simulink library "AMK_model_lib"  (R2022b)
settings: Solver=VariableStepAuto  StartTime=0.0  StopTime=10.0  RelTol=1e-3
undefined symbols (not defined in the file): DiscIntNeverNeededParam
libraries: $bdroot x15, AMK_CAN_lib x6, dspstat3 x1, slpidlib x1, simulink x1
settings Model: Creator=dr_pa  LastModifiedBy=dr_pa

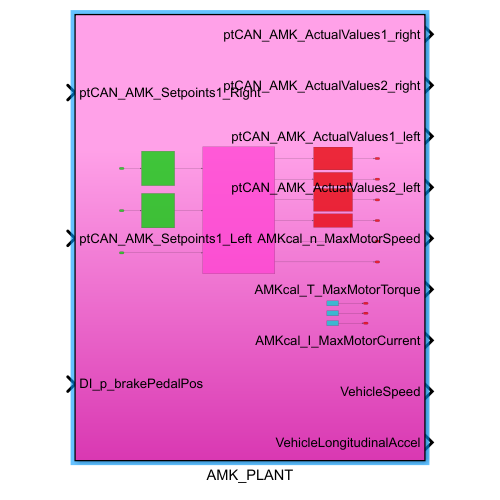
[thumbnail: Simulink's stored preview of the top-level diagram]
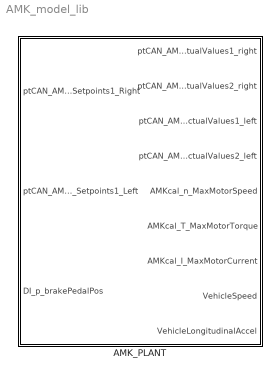
== system AMK_model_lib ==
  AMK_PLANT : Subsystem

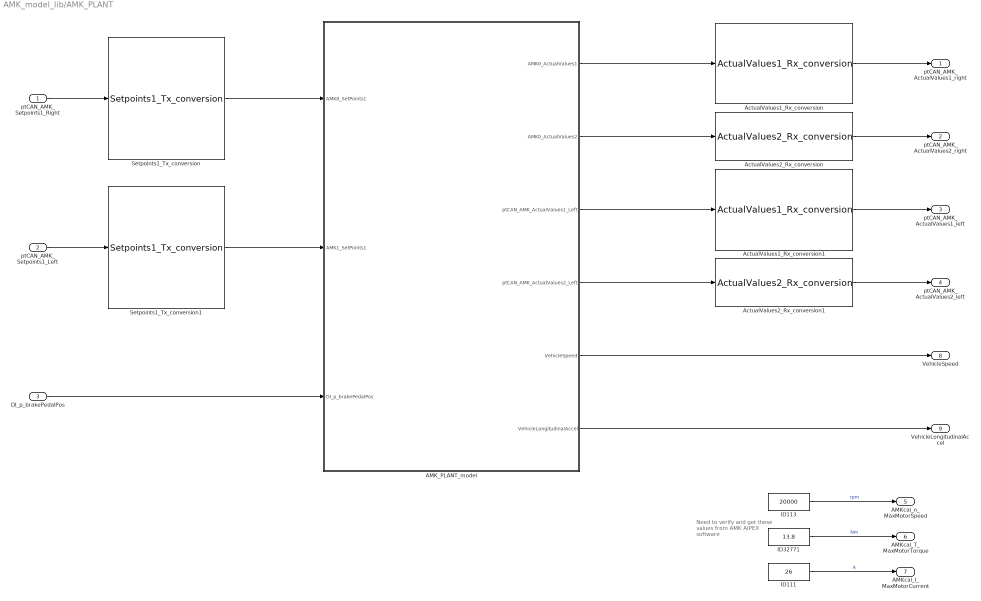
== system AMK_model_lib/AMK_PLANT ==
  note: Need to verify and get
      | these values from AMK
      | AIPEX software
  ptCAN_AMK_Setpoints1_Right : Inport
  ptCAN_AMK_Setpoints1_Left : Inport  Port=2
  DI_p_brakePedalPos : Inport  Port=3
  AMK_PLANT_model : Subsystem
  ActualValues1_Rx_conversion : AMK_CAN_lib/AMK_CAN/ActualValues1_Rx_conversion  SystemSampleTime=-1  VariantActivationTime=update diagram  Latency=0  AutoFrameSizeCalculation=off
  ActualValues1_Rx_conversion1 : AMK_CAN_lib/AMK_CAN/ActualValues1_Rx_conversion  SystemSampleTime=-1  VariantActivationTime=update diagram  Latency=0  AutoFrameSizeCalculation=off
  ActualValues2_Rx_conversion : AMK_CAN_lib/AMK_CAN/ActualValues2_Rx_conversion  SystemSampleTime=-1  VariantActivationTime=update diagram  Latency=0  AutoFrameSizeCalculation=off
  ActualValues2_Rx_conversion1 : AMK_CAN_lib/AMK_CAN/ActualValues2_Rx_conversion  SystemSampleTime=-1  VariantActivationTime=update diagram  Latency=0  AutoFrameSizeCalculation=off
  ID111 : Constant  Value=26  OutDataTypeStr=single
  ID113 : Constant  Value=20000  OutDataTypeStr=single
  ID32771 : Constant  Value=13.8  OutDataTypeStr=single
  Setpoints1_Tx_conversion : AMK_CAN_lib/AMK_CAN/Setpoints1_Tx_conversion  SystemSampleTime=-1  VariantActivationTime=update diagram  Latency=0  AutoFrameSizeCalculation=off
  Setpoints1_Tx_conversion1 : AMK_CAN_lib/AMK_CAN/Setpoints1_Tx_conversion  SystemSampleTime=-1  VariantActivationTime=update diagram  Latency=0  AutoFrameSizeCalculation=off
  ptCAN_AMK_ActualValues1_right : Outport
  ptCAN_AMK_ActualValues2_right : Outport  Port=2
  ptCAN_AMK_ActualValues1_left : Outport  Port=3
  ptCAN_AMK_ActualValues2_left : Outport  Port=4
  AMKcal_n_MaxMotorSpeed : Outport  Port=5
  AMKcal_T_MaxMotorTorque : Outport  Port=6
  AMKcal_I_MaxMotorCurrent : Outport  Port=7
  VehicleSpeed : Outport  Port=8
  VehicleLongitudinalAccel : Outport  Port=9
  wires:
  DI_p_brakePedalPos/1 -> AMK_PLANT_model/3(DI_p_brakePedalPos)
  AMK_PLANT_model/1(AMK0_ActualValues1) -> ActualValues1_Rx_conversion/1
  AMK_PLANT_model/2(AMK0_ActualValues2) -> ActualValues2_Rx_conversion/1
  AMK_PLANT_model/3(ptCAN_AMK_ActualValues1_Left) -> ActualValues1_Rx_conversion1/1
  AMK_PLANT_model/5(VehicleSpeed) -> VehicleSpeed/1
  AMK_PLANT_model/6(VehicleLongitudinalAccel) -> VehicleLongitudinalAccel/1
  Setpoints1_Tx_conversion/1 -> AMK_PLANT_model/1(AMK0_SetPoints1)
  ptCAN_AMK_Setpoints1_Right/1 -> Setpoints1_Tx_conversion/1
  Setpoints1_Tx_conversion1/1 -> AMK_PLANT_model/2(AMK1_SetPoints1)
  ptCAN_AMK_Setpoints1_Left/1 -> Setpoints1_Tx_conversion1/1
  AMK_PLANT_model/4(ptCAN_AMK_ActualValues2_Left) -> ActualValues2_Rx_conversion1/1
  ActualValues1_Rx_conversion/1 -> ptCAN_AMK_ActualValues1_right/1
  ActualValues2_Rx_conversion/1 -> ptCAN_AMK_ActualValues2_right/1
  ActualValues1_Rx_conversion1/1 -> ptCAN_AMK_ActualValues1_left/1
  ActualValues2_Rx_conversion1/1 -> ptCAN_AMK_ActualValues2_left/1
  ID113/1 -> AMKcal_n_MaxMotorSpeed/1  "rpm"
  ID32771/1 -> AMKcal_T_MaxMotorTorque/1  "Nm"
  ID111/1 -> AMKcal_I_MaxMotorCurrent/1  "A"

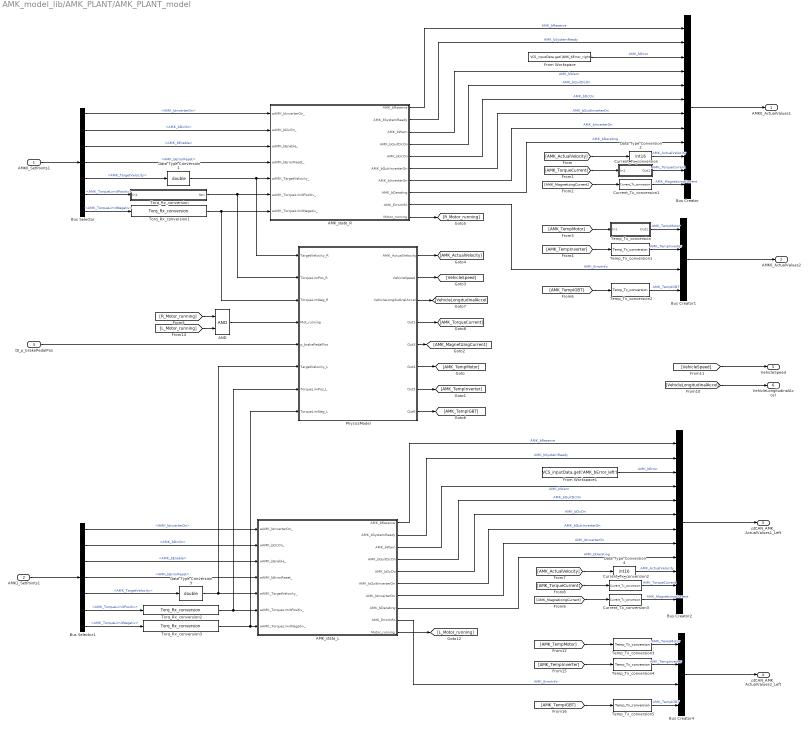
== system AMK_model_lib/AMK_PLANT/AMK_PLANT_model ==
  AMK0_SetPoints1 : Inport
  AMK1_SetPoints1 : Inport  Port=2
  DI_p_brakePedalPos : Inport  Port=3
  AMK_state_L : Stateflow chart  TreatAsAtomicUnit=on
  AMK_state_R : Stateflow chart  TreatAsAtomicUnit=on
  AND : Logic  IconShape=distinctive  AllPortsSameDT=off  OutDataTypeStr=boolean
  Bus Creator : BusCreator  Inputs=12
  Bus Creator1 : BusCreator  Inputs=4
  Bus Creator2 : BusCreator  Inputs=12
  Bus Creator4 : BusCreator  Inputs=4
  Bus Selector : BusSelector  OutputSignals=AMK_bInverterOn,AMK_bDcOn,AMK_bEnable,AMK_bErrorReset,AMK_TargetVelocity,AMK_TorqueLimitPositiv,AMK_TorqueLimitNegativ
  Bus Selector1 : BusSelector  OutputSignals=AMK_bInverterOn,AMK_bDcOn,AMK_bEnable,AMK_bErrorReset,AMK_TargetVelocity,AMK_TorqueLimitPositiv,AMK_TorqueLimitNegativ
  Current_Tx_conversion : Subsystem
  Current_Tx_conversion1 : $bdroot/AMK_PLANT/AMK_PLANT_model/Current_Tx_conversion  SystemSampleTime=-1  VariantActivationTime=update diagram  Latency=0  AutoFrameSizeCalculation=off
  Current_Tx_conversion2 : $bdroot/AMK_PLANT/AMK_PLANT_model/Current_Tx_conversion  SystemSampleTime=-1  VariantActivationTime=update diagram  Latency=0  AutoFrameSizeCalculation=off
  Current_Tx_conversion3 : $bdroot/AMK_PLANT/AMK_PLANT_model/Current_Tx_conversion  SystemSampleTime=-1  VariantActivationTime=update diagram  Latency=0  AutoFrameSizeCalculation=off
  Data Type Conversion1 : DataTypeConversion  OutDataTypeStr=double  SaturateOnIntegerOverflow=off  RndMeth=Floor
  Data Type Conversion2 : DataTypeConversion  OutDataTypeStr=int16  SaturateOnIntegerOverflow=off  RndMeth=Floor
  Data Type Conversion3 : DataTypeConversion  OutDataTypeStr=double  SaturateOnIntegerOverflow=off  RndMeth=Floor
  Data Type Conversion4 : DataTypeConversion  OutDataTypeStr=int16  SaturateOnIntegerOverflow=off  RndMeth=Floor
  From Workspace : FromWorkspace  VariableName=VCS_inputData.get('AMK_bError_right')
  From Workspace1 : FromWorkspace  VariableName=VCS_inputData.get('AMK_bError_left')
  PhysicsModel : Subsystem
  Temp_Tx_conversion : Subsystem
  Temp_Tx_conversion{1..5} (5 alike) : $bdroot/AMK_PLANT/AMK_PLANT_model/Temp_Tx_conversion  SystemSampleTime=-1  VariantActivationTime=update diagram  Latency=0  AutoFrameSizeCalculation=off
  Torq_Rx_conversion : Subsystem
  Torq_Rx_conversion1 : $bdroot/AMK_PLANT/AMK_PLANT_model/Torq_Rx_conversion  SystemSampleTime=-1  VariantActivationTime=update diagram  Latency=0  AutoFrameSizeCalculation=off
  Torq_Rx_conversion2 : $bdroot/AMK_PLANT/AMK_PLANT_model/Torq_Rx_conversion  SystemSampleTime=-1  VariantActivationTime=update diagram  Latency=0  AutoFrameSizeCalculation=off
  Torq_Rx_conversion3 : $bdroot/AMK_PLANT/AMK_PLANT_model/Torq_Rx_conversion  SystemSampleTime=-1  VariantActivationTime=update diagram  Latency=0  AutoFrameSizeCalculation=off
  AMK0_ActualValues1 : Outport
  AMK0_ActualValues2 : Outport  Port=2
  ptCAN_AMK_ActualValues1_Left : Outport  Port=3
  ptCAN_AMK_ActualValues2_Left : Outport  Port=4
  VehicleSpeed : Outport  Port=5
  VehicleLongitudinalAccel : Outport  Port=6
  wires:
  Bus Creator2/1 -> ptCAN_AMK_ActualValues1_Left/1
  Bus Creator/1 -> AMK0_ActualValues1/1
  AMK_state_R/3(AMK_bWarn) -> Bus Creator/4  "AMK_bWarn"
  Temp_Tx_conversion1/1 -> Bus Creator1/2  "AMK_TempInverter"
  PhysicsModel/1(AMK_ActualVelocity) -> [AMK_ActualVelocity]
  Data Type Conversion1/1 -> PhysicsModel/1(TargetVelocity_R), AMK_state_R/5(aAMK_TargetVelocity_)
  AMK1_SetPoints1/1 -> Bus Selector1/1
  [R_Motor_running] -> AND/1
  Current_Tx_conversion/1(Out1) -> Bus Creator/11  "AMK_TorqueCurrent"
  Data Type Conversion3/1 -> AMK_state_L/5(aAMK_TargetVelocity_), PhysicsModel/6(TargetVelocity_L)
  AMK_state_L/2(AMK_bSystemReady) -> Bus Creator2/2  "AMK_bSystemReady"
  PhysicsModel/7(Out5) -> [AMK_TempInverter]
  Current_Tx_conversion1/1 -> Bus Creator/12  "AMK_MagnetizingCurrent"
  Bus Creator4/1 -> ptCAN_AMK_ActualValues2_Left/1
  From Workspace/1 -> Bus Creator/3  "AMK_bError"
  AMK_state_R/9(AMK_ErrorInfo) -> Bus Creator1/3  "AMK_ErrorInfo"
  [AMK_TorqueCurrent] -> Current_Tx_conversion/1(In1)
  AMK_state_R/6(AMK_bQuitInverterOn) -> Bus Creator/7  "AMK_bQuitInverterOn"
  AMK_state_R/5(AMK_bDcOn) -> Bus Creator/6  "AMK_bDcOn"
  AMK_state_L/4(AMK_bQuitDcOn) -> Bus Creator2/5  "AMK_bQuitDcOn"
  AMK_state_R/10(Motor_running) -> [R_Motor_running]
  From Workspace1/1 -> Bus Creator2/3  "AMK_bError"
  PhysicsModel/2(VehicleSpeed) -> [VehicleSpeed]
  Bus Selector/3 -> AMK_state_R/3(aAMK_bEnable_)  "<AMK_bEnable>"
  AMK_state_R/8(AMK_bDerating) -> Bus Creator/9  "AMK_bDerating"
  Bus Selector/5 -> Data Type Conversion1/1  "<AMK_TargetVelocity>"
  [AMK_ActualVelocity] -> Data Type Conversion2/1
  AMK_state_L/10(Motor_running) -> [L_Motor_running]
  Torq_Rx_conversion1/1 -> PhysicsModel/3(TorqueLimNeg_R), AMK_state_R/7(aAMK_TorqueLimitNegativ_)
  Torq_Rx_conversion2/1 -> AMK_state_L/6(aAMK_TorqueLimitPositiv_), PhysicsModel/7(TorqueLimPos_L)
  AMK_state_L/5(AMK_bDcOn) -> Bus Creator2/6  "AMK_bDcOn"
  AND/1 -> PhysicsModel/4(Mot_running)
  Bus Creator1/1 -> AMK0_ActualValues2/1
  AMK_state_R/7(AMK_bInverterOn) -> Bus Creator/8  "AMK_bInverterOn"
  PhysicsModel/4(Out1) -> [AMK_TorqueCurrent]
  AMK_state_L/6(AMK_bQuitInverterOn) -> Bus Creator2/7  "AMK_bQuitInverterOn"
  Bus Selector1/1 -> AMK_state_L/1(aAMK_bInverterOn_)  "<AMK_bInverterOn>"
  PhysicsModel/8(Out6) -> [AMK_TempIGBT]
  AMK_state_L/9(AMK_ErrorInfo) -> Bus Creator4/3  "AMK_ErrorInfo"
  AMK_state_L/1(AMK_bReserve) -> Bus Creator2/1  "AMK_bReserve"
  Torq_Rx_conversion/1(Nm) -> PhysicsModel/2(TorqueLimPos_R), AMK_state_R/6(aAMK_TorqueLimitPositiv_)
  Bus Selector/2 -> AMK_state_R/2(aAMK_bDcOn_)  "<AMK_bDcOn>"
  Bus Selector1/3 -> AMK_state_L/3(aAMK_bEnable_)  "<AMK_bEnable>"
  Bus Selector1/4 -> AMK_state_L/4(aAMK_bErrorReset_)  "<AMK_bErrorReset>"
  AMK_state_L/3(AMK_bWarn) -> Bus Creator2/4  "AMK_bWarn"
  PhysicsModel/5(Out3) -> [AMK_MagnetizingCurrent]
  [L_Motor_running] -> AND/2
  DI_p_brakePedalPos/1 -> PhysicsModel/5(p_brakePedalPos)
  AMK_state_R/1(AMK_bReserve) -> Bus Creator/1  "AMK_bReserve"
  Temp_Tx_conversion/1(Out1) -> Bus Creator1/1  "AMK_TempMotor"
  Bus Selector1/5 -> Data Type Conversion3/1  "<AMK_TargetVelocity>"
  Torq_Rx_conversion3/1 -> AMK_state_L/7(aAMK_TorqueLimitNegativ_), PhysicsModel/8(TorqueLimNeg_L)
  PhysicsModel/3(VehicleLongitudinalAccel) -> [VehicleLongitudinalAccel]
  PhysicsModel/6(Out4) -> [AMK_TempMotor]
  Current_Tx_conversion3/1 -> Bus Creator2/12  "AMK_MagnetizingCurrent"
  [VehicleLongitudinalAccel] -> VehicleLongitudinalAccel/1
  Current_Tx_conversion2/1 -> Bus Creator2/11  "AMK_TorqueCurrent"
  Data Type Conversion4/1 -> Bus Creator2/10  "AMK_ActualVelocity"
  Temp_Tx_conversion2/1 -> Bus Creator1/4  "AMK_TempIGBT"
  Data Type Conversion2/1 -> Bus Creator/10  "AMK_ActualVelocity"
  [AMK_MagnetizingCurrent] -> Current_Tx_conversion1/1
  Temp_Tx_conversion3/1 -> Bus Creator4/1  "AMK_TempMotor"
  Bus Selector/4 -> AMK_state_R/4(aAMK_bErrorReset_)  "<AMK_bErrorReset>"
  AMK_state_L/8(AMK_bDerating) -> Bus Creator2/9  "AMK_bDerating"
  AMK_state_R/4(AMK_bQuitDcOn) -> Bus Creator/5  "AMK_bQuitDcOn"
  Bus Selector/1 -> AMK_state_R/1(aAMK_bInverterOn_)  "<AMK_bInverterOn>"
  Bus Selector1/2 -> AMK_state_L/2(aAMK_bDcOn_)  "<AMK_bDcOn>"
  AMK0_SetPoints1/1 -> Bus Selector/1
  Temp_Tx_conversion4/1 -> Bus Creator4/2  "AMK_TempInverter"
  AMK_state_L/7(AMK_bInverterOn) -> Bus Creator2/8  "AMK_bInverterOn"
  Temp_Tx_conversion5/1 -> Bus Creator4/4  "AMK_TempIGBT"
  AMK_state_R/2(AMK_bSystemReady) -> Bus Creator/2  "AMK_bSystemReady"
  [VehicleSpeed] -> VehicleSpeed/1
  Bus Selector/6 -> Torq_Rx_conversion/1(In1)  "<AMK_TorqueLimitPositiv>"
  Bus Selector/7 -> Torq_Rx_conversion1/1  "<AMK_TorqueLimitNegativ>"
  ? -> ?  "<AMK_TargetVelocity>"
  Bus Selector1/6 -> Torq_Rx_conversion2/1  "<AMK_TorqueLimitPositiv>"
  Bus Selector1/7 -> Torq_Rx_conversion3/1  "<AMK_TorqueLimitNegativ>"
  [AMK_TempMotor] -> Temp_Tx_conversion/1(In1)
  [AMK_TempInverter] -> Temp_Tx_conversion1/1
  [AMK_TempIGBT] -> Temp_Tx_conversion2/1
  [AMK_TempMotor] -> Temp_Tx_conversion3/1
  [AMK_TempInverter] -> Temp_Tx_conversion4/1
  [AMK_TempIGBT] -> Temp_Tx_conversion5/1
  [AMK_ActualVelocity] -> Data Type Conversion4/1
  [AMK_TorqueCurrent] -> Current_Tx_conversion2/1
  [AMK_MagnetizingCurrent] -> Current_Tx_conversion3/1

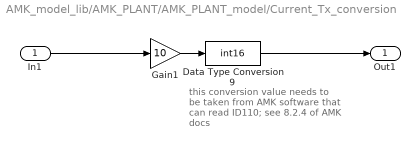
== system AMK_model_lib/AMK_PLANT/AMK_PLANT_model/Current_Tx_conversion ==
  note: this conversion value needs to be taken from AMK software that can read ID110; see 8.2.4 of AMK docs
  In1 : Inport
  Data Type Conversion9 : DataTypeConversion  OutDataTypeStr=int16  SaturateOnIntegerOverflow=off  RndMeth=Floor
  Gain1 : Gain  Gain=10
  Out1 : Outport
  wires:
  Gain1/1 -> Data Type Conversion9/1
  Data Type Conversion9/1 -> Out1/1
  In1/1 -> Gain1/1

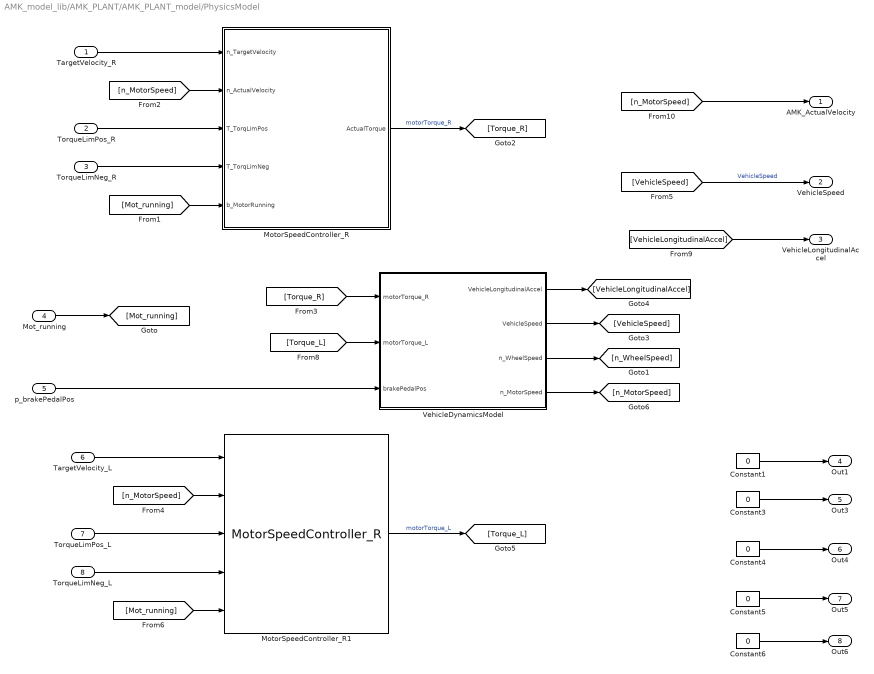
== system AMK_model_lib/AMK_PLANT/AMK_PLANT_model/PhysicsModel ==
  TargetVelocity_R : Inport
  TorqueLimPos_R : Inport  Port=2
  TorqueLimNeg_R : Inport  Port=3
  Mot_running : Inport  Port=4
  p_brakePedalPos : Inport  Port=5
  TargetVelocity_L : Inport  Port=6
  TorqueLimPos_L : Inport  Port=7
  TorqueLimNeg_L : Inport  Port=8
  Constant{1,3..6} (5 alike) : Constant  Value=0  OutDataTypeStr=single
  MotorSpeedController_R : Subsystem
  MotorSpeedController_R1 : $bdroot/AMK_PLANT/AMK_PLANT_model/PhysicsModel/MotorSpeedController_R  SystemSampleTime=-1  VariantActivationTime=update diagram  Latency=0  AutoFrameSizeCalculation=off
  VehicleDynamicsModel : Subsystem
  AMK_ActualVelocity : Outport
  VehicleSpeed : Outport  Port=2
  VehicleLongitudinalAccel : Outport  Port=3
  Out1 : Outport  Port=4
  Out3 : Outport  Port=5
  Out4 : Outport  Port=6
  Out5 : Outport  Port=7
  Out6 : Outport  Port=8
  wires:
  Mot_running/1 -> [Mot_running]
  [VehicleSpeed] -> VehicleSpeed/1  "VehicleSpeed"
  Constant3/1 -> Out3/1
  Constant4/1 -> Out4/1
  Constant5/1 -> Out5/1
  Constant6/1 -> Out6/1
  TargetVelocity_R/1 -> MotorSpeedController_R/1(n_TargetVelocity)
  TorqueLimPos_R/1 -> MotorSpeedController_R/3(T_TorqLimPos)
  TorqueLimNeg_R/1 -> MotorSpeedController_R/4(T_TorqLimNeg)
  [Mot_running] -> MotorSpeedController_R/5(b_MotorRunning)
  VehicleDynamicsModel/3(n_WheelSpeed) -> [n_WheelSpeed]
  [n_MotorSpeed] -> MotorSpeedController_R/2(n_ActualVelocity)
  MotorSpeedController_R/1(ActualTorque) -> [Torque_R]  "motorTorque_R"
  [Torque_R] -> VehicleDynamicsModel/1(motorTorque_R)
  [n_MotorSpeed] -> AMK_ActualVelocity/1
  VehicleDynamicsModel/2(VehicleSpeed) -> [VehicleSpeed]
  p_brakePedalPos/1 -> VehicleDynamicsModel/3(brakePedalPos)
  VehicleDynamicsModel/1(VehicleLongitudinalAccel) -> [VehicleLongitudinalAccel]
  MotorSpeedController_R1/1 -> [Torque_L]  "motorTorque_L"
  [n_MotorSpeed] -> MotorSpeedController_R1/2
  [Mot_running] -> MotorSpeedController_R1/5
  TorqueLimNeg_L/1 -> MotorSpeedController_R1/4
  TorqueLimPos_L/1 -> MotorSpeedController_R1/3
  TargetVelocity_L/1 -> MotorSpeedController_R1/1
  [Torque_L] -> VehicleDynamicsModel/2(motorTorque_L)
  [VehicleLongitudinalAccel] -> VehicleLongitudinalAccel/1
  VehicleDynamicsModel/4(n_MotorSpeed) -> [n_MotorSpeed]
  Constant1/1 -> Out1/1

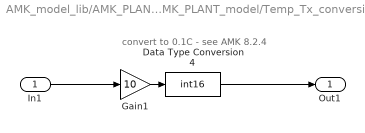
== system AMK_model_lib/AMK_PLANT/AMK_PLANT_model/Temp_Tx_conversion ==
  note: convert to 0.1C - see AMK 8.2.4
  In1 : Inport
  Data Type Conversion4 : DataTypeConversion  OutDataTypeStr=int16  SaturateOnIntegerOverflow=off  RndMeth=Floor
  Gain1 : Gain  Gain=10
  Out1 : Outport
  wires:
  Gain1/1 -> Data Type Conversion4/1
  In1/1 -> Gain1/1
  Data Type Conversion4/1 -> Out1/1

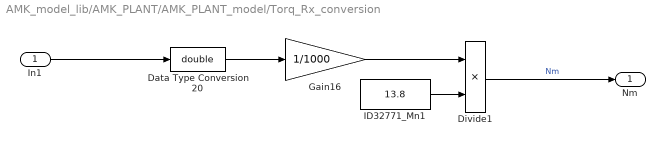
== system AMK_model_lib/AMK_PLANT/AMK_PLANT_model/Torq_Rx_conversion ==
  In1 : Inport
  Data Type Conversion20 : DataTypeConversion  OutDataTypeStr=double  SaturateOnIntegerOverflow=off  RndMeth=Floor
  Divide1 : Product  Inputs=**
  Gain16 : Gain  Gain=1/1000
  ID32771_Mn1 : Constant  Value=13.8  OutDataTypeStr=single
  Nm : Outport
  wires:
  ID32771_Mn1/1 -> Divide1/2
  Data Type Conversion20/1 -> Gain16/1
  Divide1/1 -> Nm/1  "Nm"
  Gain16/1 -> Divide1/1
  In1/1 -> Data Type Conversion20/1

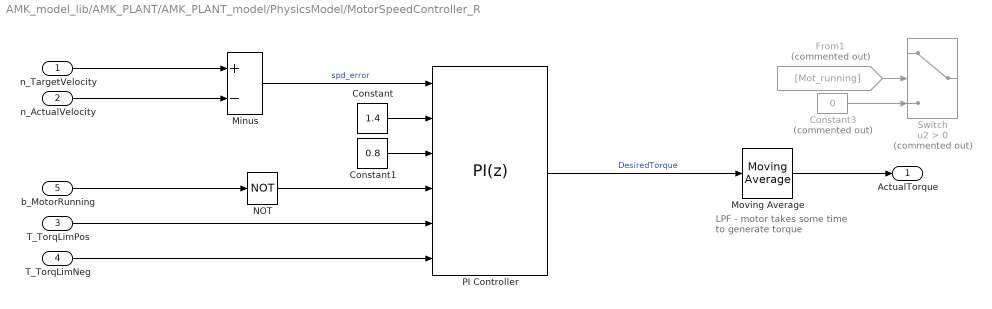
== system AMK_model_lib/AMK_PLANT/AMK_PLANT_model/PhysicsModel/MotorSpeedController_R ==
  note: LPF - motor takes some
      | time to generate torque
  n_TargetVelocity : Inport
  n_ActualVelocity : Inport  Port=2
  T_TorqLimPos : Inport  Port=3
  T_TorqLimNeg : Inport  Port=4
  b_MotorRunning : Inport  Port=5
  Constant : Constant  Value=1.4  OutDataTypeStr=single
  Constant1 : Constant  Value=0.8  OutDataTypeStr=single
  Constant3 : Constant  Commented=on  Value=0
  From1 : From  Commented=on  GotoTag=Mot_running
  Minus : Sum  Inputs=+-
  Moving Average : dspstat3/Moving Average  Method=Sliding window  ForgettingFactorPort=off  SpecifyWindowLength=on  WindowLength=5  OverlapLength=4  AllowArbitraryInputLength=off  ForgettingFactor=0.9  SimulateUsing=Code generation
  NOT : Logic  Operator=NOT  IconShape=distinctive  AllPortsSameDT=off  OutDataTypeStr=boolean
  PI Controller : slpidlib/PID Controller  Controller=PI  Form=Parallel  TimeDomain=Discrete-time  UseExternalTs=off  SampleTime=-1  IntegratorMethod=Forward Euler  FilterMethod=Forward Euler  ControllerParametersSource=external  P=1  I=1  UseKiTs=off  D=0  N=100  UseFilter=on  TunerSelectOption=Transfer Function Based (PID Tuner App)  InitialConditionSource=internal  InitialConditionForIntegrator=0  InitialConditionForFilter=0  DifferentiatorICPrevScaledInput=0  ExternalReset=level  TrackingMode=off  Kt=1  LimitOutput=on  SatLimitsSource=external  UpperSaturationLimit=1  LowerSaturationLimit=-1  LinearizeAsGain=on  AntiWindupMode=clamping  Kb=1  LimitIntegrator=off  UpperIntegratorSaturationLimit=inf  LowerIntegratorSaturationLimit=-inf  RndMeth=Simplest  POutMin=[]  POutMax=[]  IOutMin=[]  IOutMax=[]  DOutMin=[]  DOutMax=[]  NOutMin=[]  NOutMax=[]  SumOutMin=[]  SumOutMax=[]  SaturationOutDataTypeStr=single  SaturationOutMin=[]  SaturationOutMax=[]  PParamMin=[]  PParamMax=[]  IParamMin=[]  IParamMax=[]  DParamMin=[]  DParamMax=[]  NParamMin=[]  NParamMax=[]  KbParamMin=[]  KbParamMax=[]  KtParamMin=[]  KtParamMax=[]  KbOutMin=[]  KbOutMax=[]  KtOutMin=[]  KtOutMax=[]  IntegratorOutMin=[]  IntegratorOutMax=[]  FilterOutMin=[]  FilterOutMax=[]  SumI1OutMin=[]  SumI1OutMax=[]  SumI2OutMin=[]  SumI2OutMax=[]  SumI3OutMin=[]  SumI3OutMax=[]  SumI4OutMin=[]  SumI4OutMax=[]  SumDOutMin=[]  SumDOutMax=[]  DifferentiatorOutMin=[]  DifferentiatorOutMax=[]  FilterDiffOutCoefMin=[]  FilterDiffOutCoefMax=[]  ReciprocalOutMin=[]  ReciprocalOutMax=[]  SumDenOutMin=[]  SumDenOutMax=[]  SumNumOutMin=[]  SumNumOutMax=[]  DivideOutMin=[]  DivideOutMax=[]  UdiffTsProdOutMin=[]  UdiffTsProdOutMax=[]  NTsProdOutMin=[]  NTsProdOutMax=[]  UintegralTsProdOutMin=[]  UintegralTsProdOutMax=[]  UngainTsProdOutMin=[]  UngainTsProdOutMax=[]  ClampingZeroOutDataTypeStr=Inherit: Inherit via back propagation  ClampingZeroOutMin=[]  ClampingZeroOutMax=[]  FilterDenConstantOutDataTypeStr=Inherit: Inherit via back propagation  FilterDenConstantOutMin=[]  FilterDenConstantOutMax=[]  PCopyOutDataTypeStr=Inherit: Inherit via back propagation  PCopyOutMin=[]  PCopyOutMax=[]  NCopyOutDataTypeStr=Inherit: Inherit via back propagation  NCopyOutMin=[]  NCopyOutMax=[]  IntegratorContinuousStateAttributes=''  IntegratorStateMustResolveToSignalObject=off  IntegratorRTWStateStorageClass=Auto  FilterContinuousStateAttributes=''  FilterStateMustResolveToSignalObject=off  FilterRTWStateStorageClass=Auto  ParallelPVariant=ExternalParameters  IdealPVariant=Disabled  IVariant=ExternalParameters  DVariant=Disabled  IntegratorVariant=Discrete  SatVariant=External  AWVariant=DiscClampingParallel  PCopyVariant=Disabled  TRVariant=Disabled  FdbkBlocksVariant=Forward  IdealPFdbkVariant=Disabled  SatFdbkVariant=Disabled  DerivativeFilterVariant=Disabled  NVariant=Disabled  NCopyVariant=Disabled_SignalSpec  FilterICVariant=Disabled  IntegratorICVariant=InternalICs  ExternalResetVariant=ExternalReset  TRSumVariant=Passthrough  SumFdbkVariant=Disabled  SumVariant=Sum_PI  TsampFilterVariant=InternalTs  TsampNgainVariant=Passthrough  TsampIntegralVariant=Passthrough  ExternalSaturationOutDataTypeStr=single
      settings: LibrarySourceBlock=mcbhdllib/Controls/Controllers/PI Controller
  Switch : Switch  Commented=on  Criteria=u2 > Threshold  OutDataTypeStr=single  SaturateOnIntegerOverflow=off  InputSameDT=off
  ActualTorque : Outport
  wires:
  NOT/1 -> PI Controller/4
  b_MotorRunning/1 -> NOT/1
  T_TorqLimNeg/1 -> PI Controller/6
  Minus/1 -> PI Controller/1  "spd_error"
  n_TargetVelocity/1 -> Minus/1
  PI Controller/1 -> Moving Average/1  "DesiredTorque"
  Constant/1 -> PI Controller/2
  Constant1/1 -> PI Controller/3
  n_ActualVelocity/1 -> Minus/2
  From1/1 -> Switch/2
  Constant3/1 -> Switch/3
  Moving Average/1 -> ActualTorque/1
  T_TorqLimPos/1 -> PI Controller/5

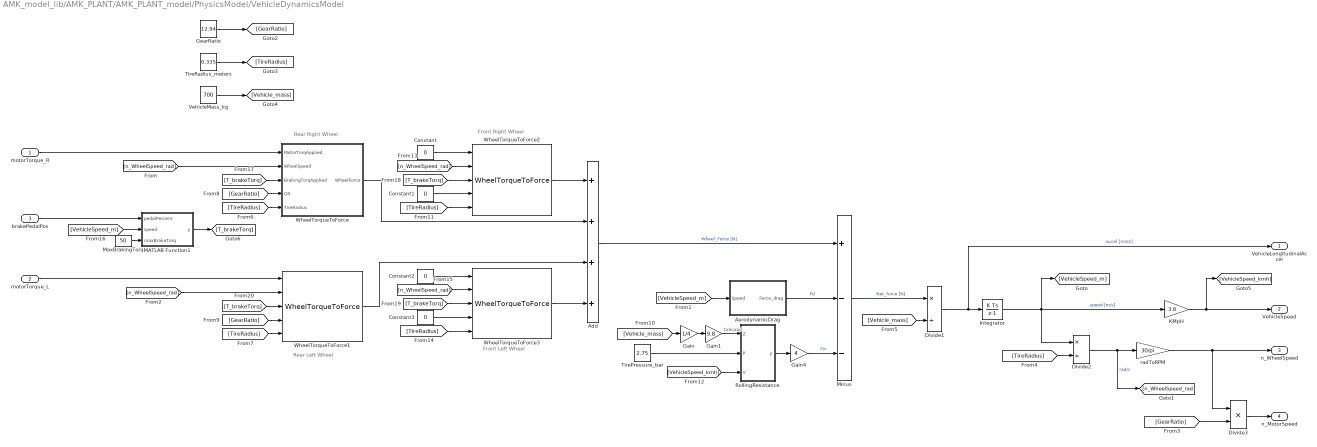
== system AMK_model_lib/AMK_PLANT/AMK_PLANT_model/PhysicsModel/VehicleDynamicsModel ==
  note: Rear Right Wheel
  note: Rear Left Wheel
  note: Front Right Wheel
  note: Front Left Wheel
  motorTorque_R : Inport
  motorTorque_L : Inport  Port=2
  brakePedalPos : Inport  Port=3
  Add : Sum  Inputs=++++
  AerodynamicDrag : Subsystem
  Constant{,1..3} (4 alike) : Constant  Value=0  OutDataTypeStr=single
  Divide1 : Product  Inputs=*/
  Divide2 : Product  Inputs=*/
  Divide3 : Product  Inputs=**
  Gain : Gain  Gain=1/4
  Gain1 : Gain  Gain=9.8
  Gain4 : Gain  Gain=4
  GearRatio : Constant  Value=12.94  OutDataTypeStr=single
  Integrator : DiscreteIntegrator  SampleTime=-1  ICPrevOutput=DiscIntNeverNeededParam  ICPrevScaledInput=DiscIntNeverNeededParam
  KMpH : Gain  Gain=3.6
  MATLAB Function1 : MATLAB Function  TreatAsAtomicUnit=on
  MaxBrakingTorq : Constant  Value=50  OutDataTypeStr=single
  Minus : Sum  Inputs=+--
  RollingResistance : MATLAB Function  TreatAsAtomicUnit=on
  TirePressure_bar : Constant  Value=2.75  OutDataTypeStr=single
  TireRadius_meters : Constant  Value=0.335  OutDataTypeStr=single
  VehicleMass_kg : Constant  Value=700  OutDataTypeStr=single
  WheelTorqueToForce : Subsystem
  WheelTorqueToForce1 : $bdroot/AMK_PLANT/AMK_PLANT_model/PhysicsModel/VehicleDynamicsModel/WheelTorqueToForce  SystemSampleTime=-1  VariantActivationTime=update diagram  Latency=0  AutoFrameSizeCalculation=off
  WheelTorqueToForce2 : $bdroot/AMK_PLANT/AMK_PLANT_model/PhysicsModel/VehicleDynamicsModel/WheelTorqueToForce  SystemSampleTime=-1  VariantActivationTime=update diagram  Latency=0  AutoFrameSizeCalculation=off
  WheelTorqueToForce3 : $bdroot/AMK_PLANT/AMK_PLANT_model/PhysicsModel/VehicleDynamicsModel/WheelTorqueToForce  SystemSampleTime=-1  VariantActivationTime=update diagram  Latency=0  AutoFrameSizeCalculation=off
  radToRPM : Gain  Gain=30/pi
  VehicleLongitudinalAccel : Outport
  VehicleSpeed : Outport  Port=2
  n_WheelSpeed : Outport  Port=3
  n_MotorSpeed : Outport  Port=4
  wires:
  radToRPM/1 -> Divide3/1, n_WheelSpeed/1
  motorTorque_R/1 -> WheelTorqueToForce/1(MotorTorqApplied)
  [n_WheelSpeed_rad] -> WheelTorqueToForce/2(WheelSpeed)
  Add/1 -> Minus/1  "Wheel_Force [N]"
  [n_WheelSpeed_rad] -> WheelTorqueToForce1/2
  motorTorque_L/1 -> WheelTorqueToForce1/1
  brakePedalPos/1 -> MATLAB Function1/1(pedalPercent)
  MaxBrakingTorq/1 -> MATLAB Function1/3(maxBrakeTorq)
  Divide1/1 -> Integrator/1, VehicleLongitudinalAccel/1  "accel [m/s2]"
  Integrator/1 -> Divide2/1, [VehicleSpeed_m], KMpH/1  "speed [m/s]"
  KMpH/1 -> [VehicleSpeed_kmh], VehicleSpeed/1
  Divide2/1 -> [n_WheelSpeed_rad], radToRPM/1  "rad/s"
  Minus/1 -> Divide1/1  "Net_force [N]"
  [VehicleSpeed_m] -> AerodynamicDrag/1(Speed)
  AerodynamicDrag/1(Force_drag) -> Minus/2  "Fd"
  GearRatio/1 -> [GearRatio]
  Divide3/1 -> n_MotorSpeed/1
  [GearRatio] -> Divide3/2
  TireRadius_meters/1 -> [TireRadius]
  VehicleMass_kg/1 -> [Vehicle_mass]
  [TireRadius] -> Divide2/2
  [Vehicle_mass] -> Divide1/2
  [TireRadius] -> WheelTorqueToForce/5(TireRadius)
  [TireRadius] -> WheelTorqueToForce1/5
  [GearRatio] -> WheelTorqueToForce/4(GR)
  [GearRatio] -> WheelTorqueToForce1/4
  [VehicleSpeed_kmh] -> RollingResistance/3(V)
  [Vehicle_mass] -> Gain/1
  Gain/1 -> Gain1/1
  Gain1/1 -> RollingResistance/1(Z)  "tireLoad"
  TirePressure_bar/1 -> RollingResistance/2(P)
  RollingResistance/1(y) -> Gain4/1
  Gain4/1 -> Minus/3  "Frr"
  Constant1/1 -> WheelTorqueToForce2/4
  WheelTorqueToForce2/1 -> Add/1
  WheelTorqueToForce/1(WheelForce) -> Add/2
  [TireRadius] -> WheelTorqueToForce2/5
  Constant/1 -> WheelTorqueToForce2/1
  [n_WheelSpeed_rad] -> WheelTorqueToForce2/2
  [TireRadius] -> WheelTorqueToForce3/5
  Constant2/1 -> WheelTorqueToForce3/1
  Constant3/1 -> WheelTorqueToForce3/4
  [n_WheelSpeed_rad] -> WheelTorqueToForce3/2
  [VehicleSpeed_m] -> MATLAB Function1/2(speed)
  WheelTorqueToForce3/1 -> Add/4
  WheelTorqueToForce1/1 -> Add/3
  MATLAB Function1/1(y) -> [T_brakeTorq]
  [T_brakeTorq] -> WheelTorqueToForce/3(BrakingTorqApplied)
  [T_brakeTorq] -> WheelTorqueToForce2/3
  [T_brakeTorq] -> WheelTorqueToForce3/3
  [T_brakeTorq] -> WheelTorqueToForce1/3

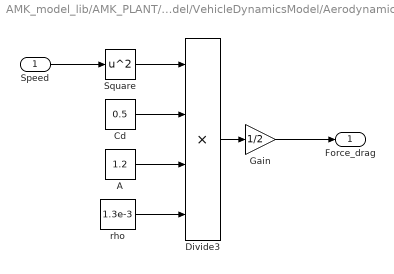
== system AMK_model_lib/AMK_PLANT/AMK_PLANT_model/PhysicsModel/VehicleDynamicsModel/AerodynamicDrag ==
  Speed : Inport
  A : Constant  Value=1.2  OutDataTypeStr=single
  Cd : Constant  Value=0.5  OutDataTypeStr=single
  Divide3 : Product  Inputs=****
  Gain : Gain  Gain=1/2
  Square : Math  Operator=square
  rho : Constant  Value=1.3e-3  OutDataTypeStr=single
  Force_drag : Outport
  wires:
  Gain/1 -> Force_drag/1
  rho/1 -> Divide3/4
  Divide3/1 -> Gain/1
  Square/1 -> Divide3/1
  A/1 -> Divide3/3
  Speed/1 -> Square/1
  Cd/1 -> Divide3/2

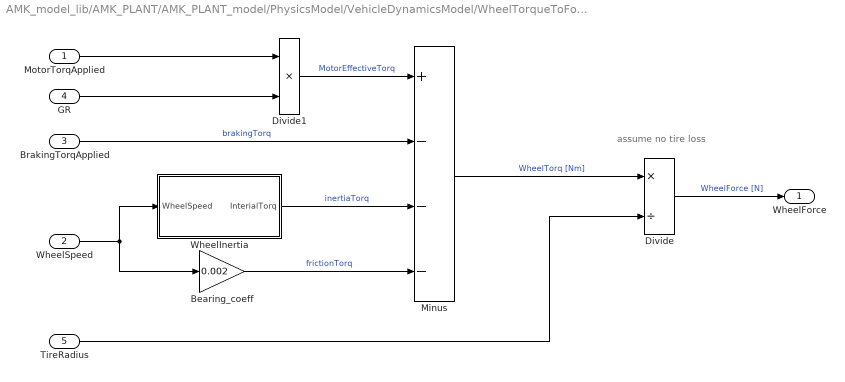
== system AMK_model_lib/AMK_PLANT/AMK_PLANT_model/PhysicsModel/VehicleDynamicsModel/WheelTorqueToForce ==
  note: assume no tire loss
  MotorTorqApplied : Inport
  WheelSpeed : Inport  Port=2
  BrakingTorqApplied : Inport  Port=3
  GR : Inport  Port=4
  TireRadius : Inport  Port=5
  Bearing_coeff : Gain  Gain=0.002
  Divide : Product  Inputs=*/
  Divide1 : Product  Inputs=**
  Minus : Sum  Inputs=+---
  WheelInertia : Subsystem
  WheelForce : Outport
  wires:
  WheelSpeed/1 -> WheelInertia/1(WheelSpeed), Bearing_coeff/1
  Minus/1 -> Divide/1  "WheelTorq [Nm]"
  WheelInertia/1(InterialTorq) -> Minus/3  "inertiaTorq"
  Divide1/1 -> Minus/1  "MotorEffectiveTorq"
  TireRadius/1 -> Divide/2
  Divide/1 -> WheelForce/1  "WheelForce [N]"
  MotorTorqApplied/1 -> Divide1/1
  BrakingTorqApplied/1 -> Minus/2  "brakingTorq"
  Bearing_coeff/1 -> Minus/4  "frictionTorq"
  GR/1 -> Divide1/2

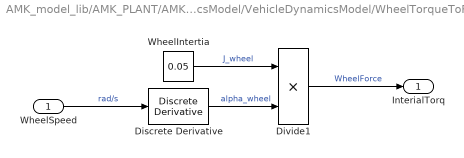
== system AMK_model_lib/AMK_PLANT/AMK_PLANT_model/PhysicsModel/VehicleDynamicsModel/WheelTorqueToForce/WheelInertia ==
  WheelSpeed : Inport
  Discrete Derivative : simulink/Discrete/Discrete Derivative  gainval=1.0  ICPrevScaledInput=0.0  OutMin=[]  OutMax=[]  OutDataType=fixdt(1, 16)  OutScaling=2^-10  DoSatur=off
  Divide1 : Product  Inputs=**
  WheelIntertia : Constant  Value=0.05  OutDataTypeStr=single
  InterialTorq : Outport
  wires:
  Discrete Derivative/1 -> Divide1/2  "alpha_wheel"
  Divide1/1 -> InterialTorq/1  "WheelForce"
  WheelSpeed/1 -> Discrete Derivative/1  "rad/s"
  WheelIntertia/1 -> Divide1/1  "J_wheel"

== stateflow chart AMK_model_lib/AMK_PLANT/AMK_PLANT_model/AMK_state_L ==
  state AMK_idle
    en:
    AMK_bReserve = 0;
    AMK_bSystemReady = 0;
    AMK_bWarn = 0;
    AMK_bQuitDcOn = 0;
    AMK_bDcOn = 0;
    AMK_bQuitInverterOn = 0;
    AMK_bInverterOn = 0;
    AMK_bDerating = 0;
    AMK_ErrorInfo = 0;
    Motor_running = false;
  note: Enable
      | en_
      | aAMK_bInverterOn_= 1
  state Startup [group]
    state Enable_System_Ready
      en:
      AMK_bSystemReady = 1;
    state Enable_Quit_Dc_On
      en:
      AMK_bQuitDcOn = 1;
      AMK_bDcOn = 1;
    state Inverter
    state Quit_Inventer_On
      en:
      AMK_bInverterOn = 1;
      AMK_bQuitInverterOn =1;
    state Motor_running
      en:
      Motor_running = true;
    Enable_System_Ready -> (junction 99) : [aAMK_bDcOn_ == 1]
    (junction 99) -> Enable_Quit_Dc_On : after(250,msec)
    Enable_Quit_Dc_On -> Inverter : [(abs(aAMK_TargetVelocity_) == 0) && ...
        | (abs(aAMK_TorqueLimitPositiv_) == 0) && ...
        | (abs(aAMK_TorqueLimitNegativ_) == 0)]
    Inverter -> (junction 101) : [(aAMK_bEnable_ == 1) && ...
        | (aAMK_bInverterOn_ == 1)]
    (junction 101) -> Quit_Inventer_On : after(250,msec)
    Quit_Inventer_On -> Motor_running
  state Shutdown [group]
    state bQuitDcOff
      en:
      AMK_bQuitDcOn = 0
    state bDcOff
      en:
      AMK_bDcOn = 0
    state Inverter_Stuff2
      % (*3) and %(*4)
    state bEnable_off
      en:
      AMK_bQuitDcOn = 0
    state bInverter_off
      en:
      AMK_bInverterOn = 0
    state Inverter_Stuff1
      % (*6)
    state Shut_off_start
    bDcOff -> bQuitDcOff
    Inverter_Stuff2 -> bDcOff : [aAMK_bDcOn_ == 0]
    bEnable_off -> Inverter_Stuff2
    bInverter_off -> bEnable_off : [aAMK_bEnable_ == 0]
    Inverter_Stuff1 -> bInverter_off : [aAMK_bInverterOn_ == 0]
    Shut_off_start -> Inverter_Stuff1
  (default) -> AMK_idle
  AMK_idle -> Enable_System_Ready : after(1,sec)
  bQuitDcOff -> Enable_System_Ready
  Motor_running -> Shut_off_start : [(aAMK_TargetVelocity_ == 0) && ...
      | (aAMK_TorqueLimitPositiv_ == 0) && ...
      | (aAMK_TorqueLimitNegativ_ == 0) && ...
      | (aAMK_bInverterOn_ == 0)]
  data: aAMK_bInverterOn_ input; aAMK_bDcOn_ input; aAMK_bEnable_ input; aAMK_bErrorReset_ input; aAMK_TargetVelocity_ input; aAMK_TorqueLimitPositiv_ input; aAMK_TorqueLimitNegativ_ input; AMK_bReserve output uint8; AMK_bSystemReady output uint8; AMK_bWarn output uint8; AMK_bQuitDcOn output uint8; AMK_bDcOn output uint8; AMK_bQuitInverterOn output uint8; AMK_bInverterOn output uint8; AMK_bDerating output uint8; AMK_ErrorInfo output int16; Motor_running output boolean =false

== matlab function AMK_model_lib/AMK_PLANT/AMK_PLANT_model/PhysicsModel/VehicleDynamicsModel/RollingResistance ==
  data: Z input; y output; P input; V input
% Tire rolling resistance Force calculator
% Z -> tire load [N]
% P -> tire pressure [bar]
% V -> vehicle speed [km/h]

function y = Frr(Z,P,V)
% define coefficients; taken from online source for a 205/75R15 97S tire
alpha = 1;
beta = -0.4;
a = 0.06;
b = 1e-4;
c = 3.7e-7;
absV = abs(V);

% equation for rolling resistance force from SAE J2452
y = Z^alpha * P^beta * (a + b*absV + c*absV^2);

% ramp to zero as V->0; multiply by sign of V to mirror the function for
% reversing
y = sign(V) * (1-exp(-absV)) * y;

== stateflow chart AMK_model_lib/AMK_PLANT/AMK_PLANT_model/AMK_state_R ==
  state AMK_idle
    en:
    AMK_bReserve = 0;
    AMK_bSystemReady = 0;
    AMK_bWarn = 0;
    AMK_bQuitDcOn = 0;
    AMK_bDcOn = 0;
    AMK_bQuitInverterOn = 0;
    AMK_bInverterOn = 0;
    AMK_bDerating = 0;
    AMK_ErrorInfo = 0;
    Motor_running = false;
  note: Enable
      | en_
      | aAMK_bInverterOn_= 1
  state Startup [group]
    state Enable_System_Ready
      en:
      AMK_bSystemReady = 1;
    state Enable_Quit_Dc_On
      en:
      AMK_bQuitDcOn = 1;
      AMK_bDcOn = 1;
    state Inverter
    state Quit_Inventer_On
      en:
      AMK_bInverterOn = 1;
      AMK_bQuitInverterOn =1;
    state Motor_running
      en:
      Motor_running = true;
    Enable_System_Ready -> (junction 99) : [aAMK_bDcOn_ == 1]
    (junction 99) -> Enable_Quit_Dc_On : after(250,msec)
    Enable_Quit_Dc_On -> Inverter : [(abs(aAMK_TargetVelocity_) == 0) && ...
        | (abs(aAMK_TorqueLimitPositiv_) == 0) && ...
        | (abs(aAMK_TorqueLimitNegativ_) == 0)]
    Inverter -> (junction 101) : [(aAMK_bEnable_ == 1) && ...
        | (aAMK_bInverterOn_ == 1)]
    (junction 101) -> Quit_Inventer_On : after(250,msec)
    Quit_Inventer_On -> Motor_running
  state Shutdown [group]
    state bQuitDcOff
      en:
      AMK_bQuitDcOn = 0
    state bDcOff
      en:
      AMK_bDcOn = 0
    state Inverter_Stuff2
      % (*3) and %(*4)
    state bEnable_off
      en:
      AMK_bQuitDcOn = 0
    state bInverter_off
      en:
      AMK_bInverterOn = 0
    state Inverter_Stuff1
      % (*6)
    state Shut_off_start
    bDcOff -> bQuitDcOff
    Inverter_Stuff2 -> bDcOff : [aAMK_bDcOn_ == 0]
    bEnable_off -> Inverter_Stuff2
    bInverter_off -> bEnable_off : [aAMK_bEnable_ == 0]
    Inverter_Stuff1 -> bInverter_off : [aAMK_bInverterOn_ == 0]
    Shut_off_start -> Inverter_Stuff1
  (default) -> AMK_idle
  AMK_idle -> Enable_System_Ready : after(1,sec)
  bQuitDcOff -> Enable_System_Ready
  Motor_running -> Shut_off_start : [(aAMK_TargetVelocity_ == 0) && ...
      | (aAMK_TorqueLimitPositiv_ == 0) && ...
      | (aAMK_TorqueLimitNegativ_ == 0) && ...
      | (aAMK_bInverterOn_ == 0)]
  data: aAMK_bInverterOn_ input; aAMK_bDcOn_ input; aAMK_bEnable_ input; aAMK_bErrorReset_ input; aAMK_TargetVelocity_ input; aAMK_TorqueLimitPositiv_ input; aAMK_TorqueLimitNegativ_ input; AMK_bReserve output uint8; AMK_bSystemReady output uint8; AMK_bWarn output uint8; AMK_bQuitDcOn output uint8; AMK_bDcOn output uint8; AMK_bQuitInverterOn output uint8; AMK_bInverterOn output uint8; AMK_bDerating output uint8; AMK_ErrorInfo output int16; Motor_running output boolean =false

== matlab function AMK_model_lib/AMK_PLANT/AMK_PLANT_model/PhysicsModel/VehicleDynamicsModel/MATLAB Function1 ==
  data: pedalPercent input; y output; speed input; maxBrakeTorq input
% Braking force model, based on a shifted sigmoid function
% this model is dumb, but at least it correctly models F_brake = 0 @ 0km/h
% and is mirrored for speed>0 and speed<0

function y = Fb(pedalPercent, speed, maxBrakeTorq)

y = pedalPercent * (2*maxBrakeTorq/(1 + exp(-speed/2)) - maxBrakeTorq);
